simulink model "PIDController_theta1"  (R2022a)
settings: Solver=ode5  StartTime=0.0  StopTime=0.0036988  FixedStep=9.2471e-05  RelTol=1e-3
settings Model: Creator=Admin  LastModifiedBy=mquyet
settings SolverCC: AlgebraicLoopSolver=TrustRegion
settings DataIOCC: ReturnWorkspaceOutputs=off
settings DebuggingCC: UnconnectedInputMsg=warning  UnconnectedOutputMsg=warning  UnconnectedLineMsg=warning  SFMachineParentedDataDiag=warning  ArithmeticOperatorsInVariantConditions=warning
settings SFSimCC: SimUseLocalCustomCode=off  CustomCodeUndefinedFunction=UseInterfaceOnly
settings RTWCC: RTWUseLocalCustomCode=off
settings CodeAppCC: StateflowObjectComments=on

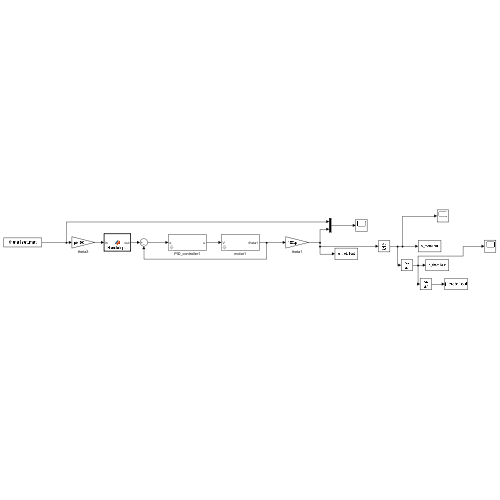
[thumbnail: Simulink's stored preview of the top-level diagram]
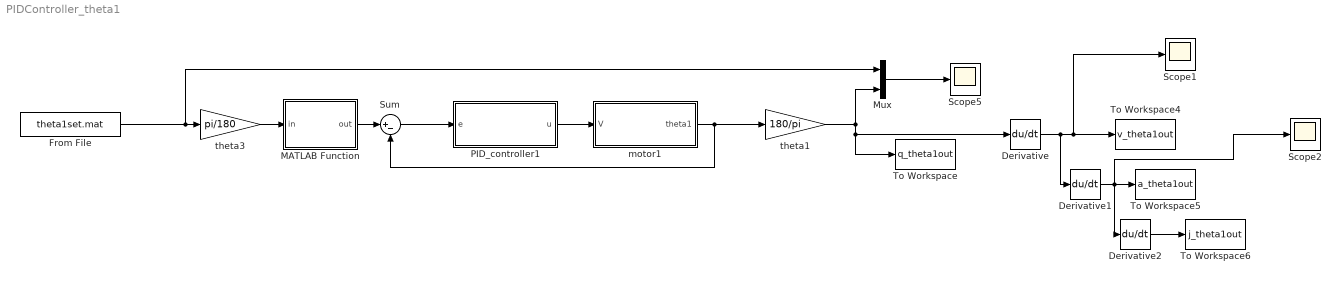
== system PIDController_theta1 ==
  Derivative : Derivative
  Derivative1 : Derivative
  Derivative2 : Derivative
  From File : FromFile  FileName=theta1set.mat
  MATLAB Function : MATLAB Function  TreatAsAtomicUnit=on
  Mux : Mux  Inputs=2
  PID_controller1 : Subsystem  mask{Kp=800, Ki=100, Kd=5}
  Scope1 : Scope
  Scope2 : Scope
  Scope5 : Scope
  Sum : Sum  Inputs=|+-
  To Workspace : ToWorkspace  VariableName=q_theta1out  SampleTime=-1
  To Workspace4 : ToWorkspace  VariableName=v_theta1out  SampleTime=-1
  To Workspace5 : ToWorkspace  VariableName=a_theta1out  SampleTime=-1
  To Workspace6 : ToWorkspace  VariableName=j_theta1out  SampleTime=-1
  motor1 : Subsystem  mask{Ki=0.1, Kb=0.1, L=0.5, R=2, Jeff=0.02, Beff=0.2, N=100}
  theta1 : Gain  Gain=180/pi
  theta3 : Gain  Gain=pi/180
  wires:
  Sum/1 -> PID_controller1/1(e)
  PID_controller1/1(u) -> motor1/1(V)
  theta1/1 -> To Workspace/1, Derivative/1, Mux/2
  motor1/1(theta1) -> theta1/1, Sum/2
  MATLAB Function/1(out) -> Sum/1
  Derivative/1 -> Derivative1/1, Scope1/1, To Workspace4/1
  Derivative1/1 -> Scope2/1, Derivative2/1, To Workspace5/1
  Derivative2/1 -> To Workspace6/1
  From File/1 -> Mux/1, theta3/1
  Mux/1 -> Scope5/1
  theta3/1 -> MATLAB Function/1(in)

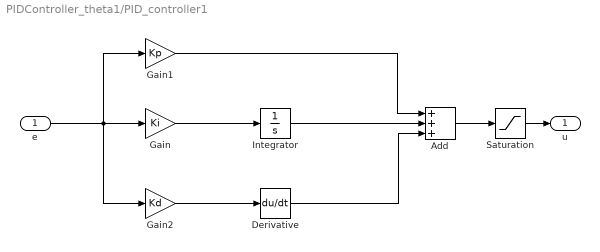
== system PIDController_theta1/PID_controller1 ==
  e : Inport
  Add : Sum  Inputs=+++
  Derivative : Derivative
  Gain : Gain  Gain=Ki
  Gain1 : Gain  Gain=Kp
  Gain2 : Gain  Gain=Kd
  Integrator : Integrator
  Saturation : Saturate  UpperLimit=300  LowerLimit=-300
  u : Outport  VectorParamsAs1DForOutWhenUnconnected=off
  wires:
  e/1 -> Gain2/1, Gain1/1, Gain/1
  Gain/1 -> Integrator/1
  Gain2/1 -> Derivative/1
  Gain1/1 -> Add/1
  Integrator/1 -> Add/2
  Derivative/1 -> Add/3
  Add/1 -> Saturation/1
  Saturation/1 -> u/1

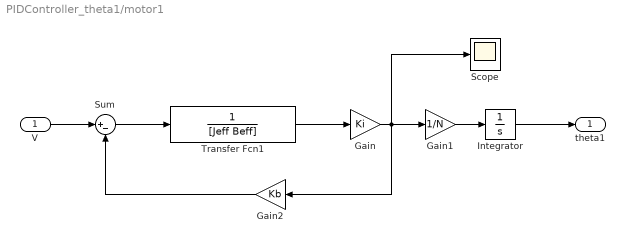
== system PIDController_theta1/motor1 ==
  V : Inport
  Gain : Gain  Gain=Ki
  Gain1 : Gain  Gain=1/N
  Gain2 : Gain  Gain=Kb
  Integrator : Integrator  InitialCondition=-85.1512
  Scope : Scope
  Sum : Sum  Inputs=|+-
  Transfer Fcn1 : TransferFcn  Denominator=[Jeff Beff]
  theta1 : Outport  VectorParamsAs1DForOutWhenUnconnected=off
  wires:
  Transfer Fcn1/1 -> Gain/1
  Gain2/1 -> Sum/2
  V/1 -> Sum/1
  Sum/1 -> Transfer Fcn1/1
  Gain/1 -> Gain1/1, Gain2/1, Scope/1
  Gain1/1 -> Integrator/1
  Integrator/1 -> theta1/1

== matlab function PIDController_theta1/MATLAB Function ==
  settings: updateMethod=DISCRETE
  data: in input; out output
function out = HandleInput(in)

out = in
persistent pre
if isempty(pre)
    pre = 0;
end

while (out - pre > 1.5*pi)
    out = out - 2*pi;
end

while (out - pre < -1.5*pi)
    out = out + 2*pi;
end
